simulink model "Buck_Converter_Closed_Loop"  (R2025a)
settings: Solver=FixedStepAuto  StartTime=0.0  StopTime=inf  RelTol=1e-3  EnableMultiTasking=on
libraries: spsSeriesRLCBranchLib x3, stm32f4xxblockslib x2, spsDCVoltageSourceLib x1, spsDiodeLib x1, spsGroundLib x1, spsMosfetLib x1, spsPWMGeneratorDCDCLib x1, peripheralslib x1, stm32blockslib x1, spsVoltageMeasurementLib x1, sps_lib x1
settings Model: STM32="{\"AnalogOutput\":{\"ID\":\"Buck_Converter_Closed_Loop:3\"},\"AnalogInput\":{\"ID\":\"Buck_Converter_Closed_Loop:11\"},\"PWMOutput\":{\"ID\":\"Buck_Converter_Closed_Loop:12\"}}"  Creator=GNKRISHNAN  LastModifiedBy=GNKRISHNAN
settings SolverCC: AutoInsertRateTranBlk=on
settings OptimizationCC: DefaultParameterBehavior=Inlined  EnhancedBackFolding=on  BooleansAsBitfields=on  PassReuseOutputArgsAs=Individual arguments  StateBitsets=on  DataBitsets=on  ZeroExternalMemoryAtStartup=off  ZeroInternalMemoryAtStartup=off  MaxStackSize=512  DifferentSizesBufferReuse=on  OptimizationPriority=RAM  OptimizationCustomize=off  EfficientTunableParamExpr=on
settings DebuggingCC: ParameterTunabilityLossMsg=error
settings HardwareCC: ProdBitPerPointer=32.0  ProdBitPerSizeT=32.0  ProdBitPerPtrDiffT=32.0  ProdLargestAtomicInteger=Long  ProdLargestAtomicFloat=Double  ProdWordSize=32.0  ProdLongLongMode=on  ProdHWDeviceType=ARM Compatible->ARM Cortex-M
settings SFSimCC: MATLABDynamicMemAlloc=off
settings RTWCC: SystemTargetFile=ert.tlc  HardwareBoard=STM32G4xx Based  TemplateMakefile=ert_default_tmf  Toolchain=GNU Tools for ARM Embedded Processors  Description=Embedded Coder
settings CodeAppCC: ForceParamTrailComments=on  IgnoreCustomStorageClasses=off  OperatorAnnotations=on  SimulinkDataObjDesc=on  SFDataObjDesc=on  InsertBlockDesc=on
settings ERTTargetCC: ExtModeTransport=3.0  ExtModeStaticAllocSize=2048.0  TargetLangStandard=C99 (ISO)  CodeReplacementLibrary=ARM Cortex-M  SupportContinuousTime=on  InstructionSetFMA=on

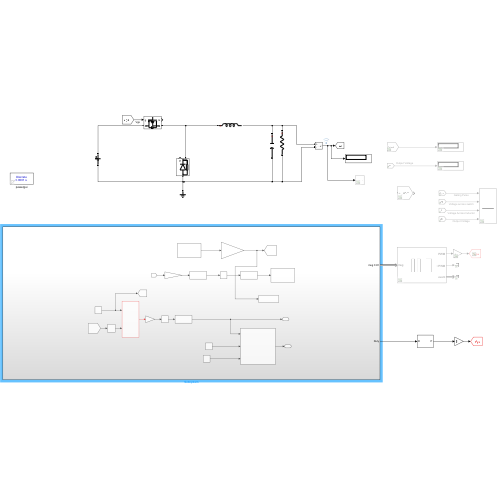
[thumbnail: Simulink's stored preview of the top-level diagram]
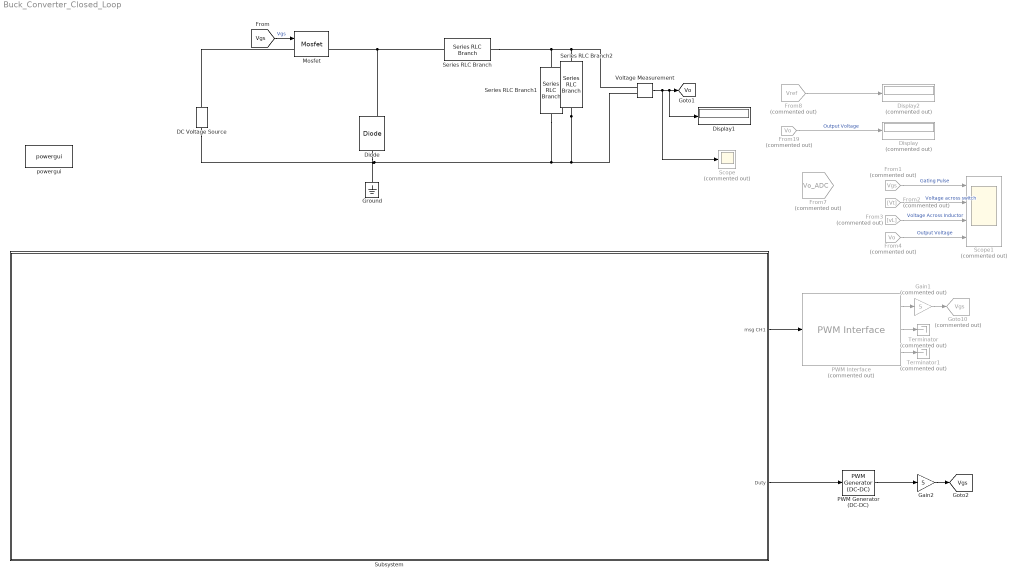
== system Buck_Converter_Closed_Loop ==
  DC Voltage Source : spsDCVoltageSourceLib/DC Voltage Source  Amplitude=100  Measurements=None
  Diode : spsDiodeLib/Diode  Ron=0.001  Lon=0  Vf=0.8  IC=0  UseSnubber=0  Rs=500  Cs=250e-9  Measurements=on
  Display : Display  Commented=on
  Display1 : Display
  Display2 : Display  Commented=on
  From1 : From  Commented=on  GotoTag=Vgs  TagVisibility=global
  From19 : From  Commented=on  GotoTag=Vo  TagVisibility=global
  From2 : From  Commented=on  GotoTag=Vt  TagVisibility=global
  From3 : From  Commented=on  GotoTag=vL  TagVisibility=global
  From4 : From  Commented=on  GotoTag=Vo  TagVisibility=global
  From7 : From  Commented=on  GotoTag=Vo_ADC  TagVisibility=global
  From8 : From  Commented=on  GotoTag=Vref  TagVisibility=global
  Gain1 : Gain  Commented=on  Gain=5
  Gain2 : Gain  Gain=5
  Goto10 : Goto  Commented=on  GotoTag=Vgs  TagVisibility=global
  Ground : spsGroundLib/Ground  LConnTagsString=a
  Mosfet : spsMosfetLib/Mosfet  Ron=0.1  Lon=0  Rd=0.01  Vfd=1.2  IC=0  Rs=1e5  Cs=inf  Measurements=on
  PWM Generator (DC-DC) : spsPWMGeneratorDCDCLib/PWM Generator (DC-DC)  Fsw=40e3  Ts=0
  PWM Interface : peripheralslib/PWM Interface  Commented=on  Period=1/(40e3)  OutSigMode=Switching  CounterMode=Up  GenCompPWM=on  DeadTimeTopPWM=1e-6  DeadTimeBottomPWM=1e-6  EventCondition2=End of PWM period  DataType=double  PWMAtStartPeriod=High  PWMAtMidPeriod=NoChange  PWMAtCMP1=Low  PWMAtCMP1UpCnt=Low  PWMAtCMP1DwnCnt=High  PWMAtCMP2=NoChange  PWMAtCMP2UpCnt=NoChange  PWMAtCMP2DwnCnt=NoChange  OutCountDir=off  PhaseOffset=0  EventType=ADC start  EventCondition1=End of PWM period  NumADCSOCToWait=1st event  NumADCSOCReplica=1  InterruptCond=End of PWM period  IntLatency=0  NumInterruptToWait=1st event
      settings: SamplingMode=Immediate (at compare matches)
  Scope : Scope  Commented=on
  Scope1 : Scope  Commented=on  NumInputPorts=4
      settings: ActiveDisplayYMinimum=-0.62499999999999989  ActiveDisplayYMaximum=5.625  DataLoggingVariableName=ScopeData4
  Series RLC Branch : spsSeriesRLCBranchLib/Series RLC Branch  LConnTagsString=__new0  RConnTagsString=__new0  BranchType=L  Resistance=1  Inductance=150e-6  SetiL0=off  InitialCurrent=0  Capacitance=1e-6  Setx0=off  InitialVoltage=0  Measurements=None
  Series RLC Branch1 : spsSeriesRLCBranchLib/Series RLC Branch  LConnTagsString=__new0  RConnTagsString=__new0  BranchType=C  Resistance=1  Inductance=150e-6  SetiL0=off  InitialCurrent=0  Capacitance=10e-6  Setx0=off  InitialVoltage=0  Measurements=None
  Series RLC Branch2 : spsSeriesRLCBranchLib/Series RLC Branch  LConnTagsString=__new0  RConnTagsString=__new0  BranchType=R  Resistance=10  Inductance=150e-6  SetiL0=off  InitialCurrent=0  Capacitance=1e-6  Setx0=off  InitialVoltage=0  Measurements=None
  Subsystem : Subsystem
  Terminator : Terminator  Commented=on
  Terminator1 : Terminator  Commented=on
      settings: InputPortMessageModes=m
  Voltage Measurement : spsVoltageMeasurementLib/Voltage Measurement  PhasorSimulation=off  OutputType=Complex  PSBequivalent=0
  powergui : sps_lib/powergui  Priority=1  SimulationMode=Discrete  SampleTime=1e-4  frequency=60  Iterations=50  frequencyindice=0  Pbase=100e6  ErrMax=1e-4  UnitsV=kV  UnitsW=MW  buscounter=0  FunctionMessages=off  echomessages=off  EnableUseOfTLC=off  CurrentSourceSwitches=off  DisableSnubberDevices=off  DisableRonSwitches=off  DisableVfSwitches=off  DisplayEquations=off  AutomaticDiscreteSolvers=off  SolverType=Tustin/Backward Euler (TBE)  Interpol=off  ExternalGateDelay=off  methode=off  Ts=100  x0status=blocks  SPID=on  SwTol=0  HookPort=off  NonlinearTolerance=1e-4  nMaxIteration=100  ContinueOnMaxIteration=off  RestoreLinks=warning  ResistiveCurrentMeasurement=off  Frange=[0:2:500]  Ylog=off  Xlog=on  ShowGrid=off  save=off  variable=ZData  structure=0  ZoomFFT=off  StartTime=0.0  cycles=1  DisplayStyle=1  fundamental=60  FreqAxis=off  MaxFrequency=1000  frequencyindicesteady=1  RmsSteady=1  display=off
  tag scope: Vgs=global, Vo=global
  wires:
  From19/1 -> Display/1  "Output Voltage"
  From4/1 -> Scope1/4  "Output Voltage"
  From1/1 -> Scope1/1  "Gating Pulse"
  From2/1 -> Scope1/2  "Voltage across switch"
  From3/1 -> Scope1/3  "Voltage Across Inductor"
  From8/1 -> Display2/1
  PWM Interface/1 -> Gain1/1
  Gain1/1 -> Goto10/1
  PWM Interface/2 -> Terminator/1
  PWM Interface/3 -> Terminator1/1
  Subsystem/1(msg CH1) -> PWM Interface/1
  Gain2/1 -> [Vgs]
  Subsystem/2(Duty) -> PWM Generator (DC-DC)/1
  PWM Generator (DC-DC)/1 -> Gain2/1
  Voltage Measurement/1 -> Scope/1, Display1/1, [Vo]
  [Vgs] -> Mosfet/1  "Vgs"
  connections:
  Voltage Measurement/LConn1 -- Series RLC Branch1/LConn1 -- Series RLC Branch/RConn1 -- Series RLC Branch2/LConn1
  Diode/RConn1 -- Series RLC Branch/LConn1 -- Mosfet/RConn1
  Series RLC Branch2/RConn1 -- Voltage Measurement/LConn2 -- Series RLC Branch1/RConn1 -- Ground/LConn1 -- DC Voltage Source/LConn1 -- Diode/LConn1
  DC Voltage Source/RConn1 -- Mosfet/LConn1

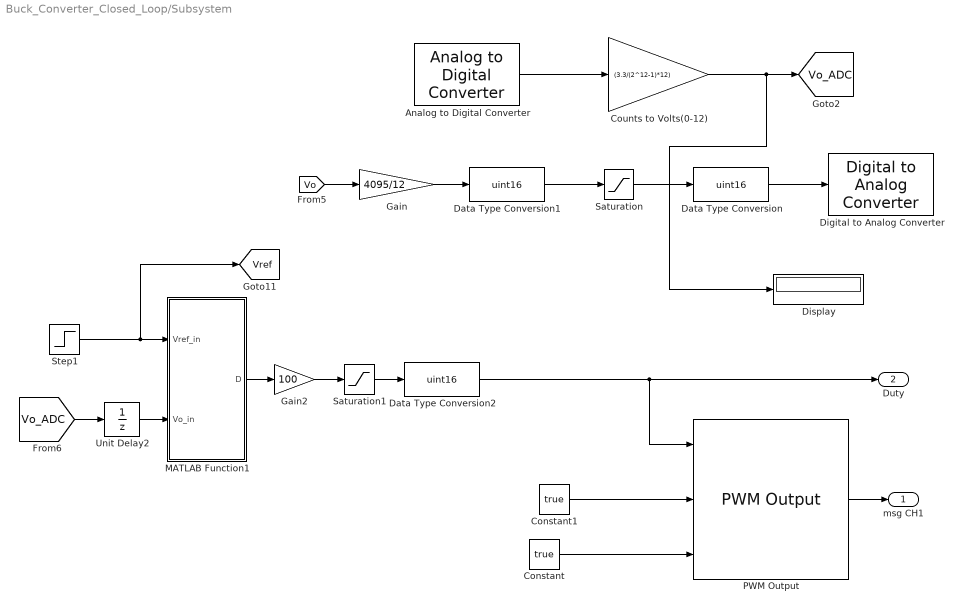
== system Buck_Converter_Closed_Loop/Subsystem ==
  Analog to Digital Converter : stm32f4xxblockslib/Analog to Digital Converter  ADCModule=ADC1  ConversionGroup=Regular  TriggerMode=Trigger and read  NumberOfConversions=1  EnableBufferConv=off  BufferLength=1  OutputStatus=off  SampleTime=-1  EnableSimPort=off  hoistedMaskSrc=ECSoC/ECSimCodegen/Analog to Digital Converter
  Constant : Constant  Value=true
  Constant1 : Constant  Value=true
  Counts to Volts(0-12) : Gain  Gain=(3.3/(2^12-1)*12)  ParamDataTypeStr=single
  Data Type Conversion : DataTypeConversion  OutDataTypeStr=uint16  SaturateOnIntegerOverflow=off  RndMeth=Floor
  Data Type Conversion1 : DataTypeConversion  OutDataTypeStr=uint16  SaturateOnIntegerOverflow=off  RndMeth=Floor
  Data Type Conversion2 : DataTypeConversion  OutDataTypeStr=uint16  SaturateOnIntegerOverflow=off  RndMeth=Floor
  Digital to Analog Converter : stm32blockslib/Digital to Analog Converter  DACModule=DAC1  TriggerType=Write only  ChannelGroup=Channel1  waveGenEnable=off  waveType=Noise/Triangular  TriggerEnable=on  stepTriggerEnable=on  resetTriggerEnable=on  TrigConfig=Independent trigger  DataLength=12 bits  DataAlignment=Right alignment  dacEnable=off  OutputStatus=off
      settings: LibrarySourceBlock=stm32g4xxblockslib/Digital to Analog Converter
  Display : Display
  Gain : Gain  Gain=4095/12
  Gain2 : Gain  Gain=100
  MATLAB Function1 : MATLAB Function  TreatAsAtomicUnit=on
  PWM Output : stm32f4xxblockslib/PWM Output  ProcessorFamily=STM32G4  TimerModule=TIM1  DutycycleUnits=Percentage  EnableChannel1=on  EnableCaptureCompare1Input=off  EnableCaptureCompare1ComplementaryInput=off  EnableOutputCompare1ModeInput=off  EnableChannel2=off  EnableCaptureCompare2Input=off  EnableCaptureCompare2ComplementaryInput=off  EnableOutputCompare2ModeInput=off  EnableChannel3=off  EnableCaptureCompare3Input=off  EnableCaptureCompare3ComplementaryInput=off  EnableOutputCompare3ModeInput=off  EnableChannel4=off  EnableCaptureCompare4Input=off  EnableCaptureCompare4ComplementaryInput=off  EnableOutputCompare4ModeInput=off  EnableChannel5=off  EnableCaptureCompare5Input=off  EnableOutputCompare5ModeInput=off  EnableChannel6=off  EnableCaptureCompare6Input=off  EnableOutputCompare6ModeInput=off  EnableCounterInput=on  EnableMainOutputInput=on  EnableFrequencyInput=off  SetRCAfterCE=off  OutputDirection=off  OutputMainOutputEnableStatus=off  SampleTime=0.1  EnableSimPort=on  EnableUpdateEvent=off  EnableCaptureCompare1Event=off  EnableCaptureCompare2Event=off  EnableCaptureCompare3Event=off  EnableCaptureCompare4Event=off  EnableTriggerEvent=off  EnableBreakEvent=off  EnableBreakEvent2=off  hoistedMaskSrc=ECSoC/ECSimCodegen/PWM Output
      settings: LibrarySourceBlock=stm32g4xxblockslib/PWM Output
  Saturation : Saturate  UpperLimit=4095  LowerLimit=0
  Saturation1 : Saturate  UpperLimit=100  LowerLimit=0
  Step1 : Step  Time=15  Before=8  After=4.5  SampleTime=1/(40e3)
  Unit Delay2 : UnitDelay  SampleTime=-1  HasFrameUpgradeWarning=on
  msg CH1 : Outport
  Duty : Outport  Port=2
  tag scope: Vo_ADC=global, Vref=global
  wires:
  Data Type Conversion/1 -> Digital to Analog Converter/1
  Step1/1 -> [Vref], MATLAB Function1/1(Vref_in)
  Constant/1 -> PWM Output/3
  Data Type Conversion2/1 -> Duty/1, PWM Output/1
  Data Type Conversion1/1 -> Saturation/1
  Analog to Digital Converter/1 -> Counts to Volts(0-12)/1
  [Vo_ADC] -> Unit Delay2/1
  Unit Delay2/1 -> MATLAB Function1/2(Vo_in)
  Constant1/1 -> PWM Output/2
  Gain/1 -> Data Type Conversion1/1
  Gain2/1 -> Saturation1/1
  Saturation/1 -> Data Type Conversion/1
  Saturation1/1 -> Data Type Conversion2/1
  MATLAB Function1/1(D) -> Gain2/1
  [Vo] -> Gain/1
  PWM Output/1 -> msg CH1/1
  Counts to Volts(0-12)/1 -> Display/1, [Vo_ADC]

== matlab function Buck_Converter_Closed_Loop/Subsystem/MATLAB Function1 ==
  data: Vref_in input; D output; Vo_in input
function D = buck_controller(Vref_in, Vo_in)
%#codegen
% Single-loop Voltage Mode PI Controller for STM32
% Plant: L = 150uH, C = 10uF, fs = 40kHz

%% -------- Hardware Constants (Single Precision) --------
persistent is_initialized
persistent int_v

% Controller Gains
Kp = single(0.025); 
Ki = single(80.0);
Ts = single(1/40000);

% Pre-calculated Discrete Gain to save one cycle: Ki_step = Ki * Ts
Ki_step = single(0.002); 

Dmax = single(0.95);
Dmin = single(0.0);

%% -------- Initialization --------
if isempty(is_initialized)
    int_v = single(0.0);
    is_initialized = true;
end

%% -------- Type Casting Inputs --------
% Ensure inputs from ADC/Simulink are treated as single
Vref = single(Vref_in);
Vo = single(Vo_in);

%% -------- Voltage Control Loop --------
ev = Vref - Vo;

% Calculate potential duty cycle
% Using pre-calculated Ki_step (Ki * Ts)
D_unclamped = (Kp * ev) + int_v;

%% -------- Saturation & Anti-windup (Clamping) --------
% We use a conditional clamping strategy for better C-code generation
if D_unclamped > Dmax
    D = Dmax;
elseif D_unclamped < Dmin
    D = Dmin;
else
    D = D_unclamped;
    % Only update integrator if output is NOT saturated (Clamping)
    int_v = int_v + (ev * Ki_step);
end

end
